simulink model "humanFollower1"  (R2018b)
settings: Solver=VariableStepAuto  StartTime=0.0  StopTime=inf  MaxStep=0.2  MinStep=0.2  RelTol=1e-3
undefined symbols (not defined in the file or in its folder): Angular, Linear
libraries: robotlib x8
settings Model: Creator=ckreienk  LastModifiedBy=ckreienk
settings SolverCC: InitialStep=0.2

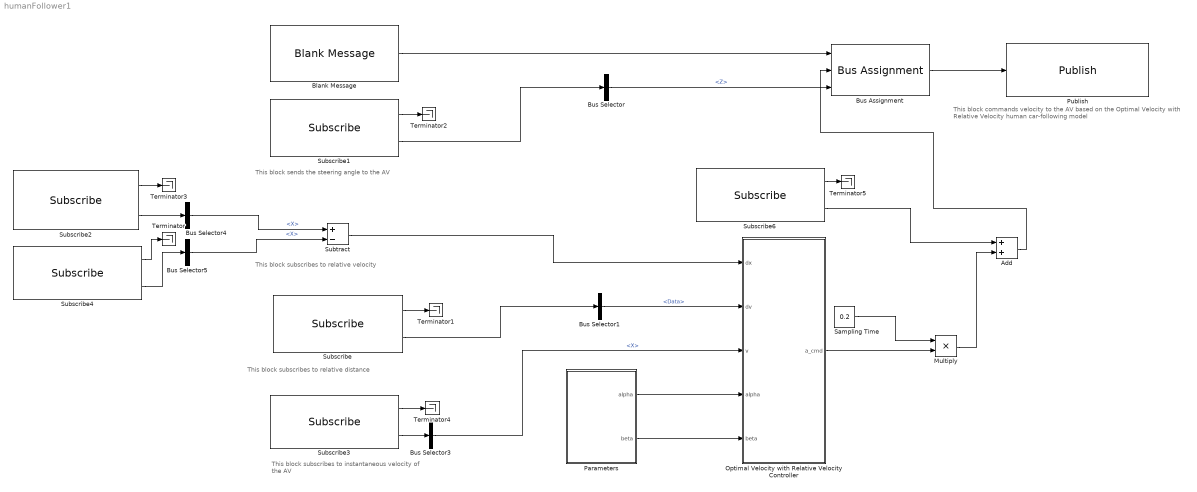
== system humanFollower1 ==
  note: This block sends the steering angle
      | to the AV
  note: This block subscribes to relative velocity
  note: This block subscribes to relative distance
  note: This block subscribes to
      | instantaneous velocity of the AV
  note: This block commands velocity to the AV based
      | on the Optimal Velocity with Relative Velocity
      | human car-following model
  Add : Sum
  Blank Message : robotlib/Blank Message  messageClass=Message  entityType=geometry_msgs/Twist  messageType=geometry_msgs/Twist  SampleTime=inf
      settings: SourceProductBaseCode=RO
  Bus Assignment : BusAssignment  AssignedSignals=Linear.X,Angular.Z
  Bus Selector : BusSelector  OutputSignals=Angular.Z
  Bus Selector1 : BusSelector  OutputSignals=Data
  Bus Selector3 : BusSelector  OutputSignals=Linear.X
  Bus Selector4 : BusSelector  OutputSignals=Linear.X
  Bus Selector5 : BusSelector  OutputSignals=Linear.X
  Multiply : Product
  Optimal Velocity with Relative Velocity Controller : Subsystem
  Parameters : Subsystem
  Publish : robotlib/Publish  topicSource=Select from ROS network  topic=/followerVehicle/cmd_vel  messageType=geometry_msgs/Twist  messageQueueLength=1
      settings: SourceProductBaseCode=RO
  Sampling Time : Constant  Value=0.2
  Subscribe : robotlib/Subscribe  topicSource=Select from ROS network  topic=/followerVehicle/distanceEstimatorSteeringBased/dist  messageType=std_msgs/Float64  sampleTime=-1  messageQueueLength=1
      settings: SourceProductBaseCode=RO
  Subscribe1 : robotlib/Subscribe  topicSource=Select from ROS network  topic=/leadVehicle/cmd_vel  messageType=geometry_msgs/Twist  sampleTime=-1  messageQueueLength=1
      settings: SourceProductBaseCode=RO
  Subscribe2 : robotlib/Subscribe  topicSource=Select from ROS network  topic=/leadVehicle/cmd_vel  messageType=geometry_msgs/Twist  sampleTime=-1  messageQueueLength=1
      settings: SourceProductBaseCode=RO
  Subscribe3 : robotlib/Subscribe  topicSource=Select from ROS network  topic=/followerVehicle/cmd_vel  messageType=geometry_msgs/Twist  sampleTime=-1  messageQueueLength=1
      settings: SourceProductBaseCode=RO
  Subscribe4 : robotlib/Subscribe  topicSource=Select from ROS network  topic=/followerVehicle/cmd_vel  messageType=geometry_msgs/Twist  sampleTime=-1  messageQueueLength=1
      settings: SourceProductBaseCode=RO
  Subscribe6 : robotlib/Subscribe  topicSource=Select from ROS network  topic=/followerVehicle/cmd_vel  messageType=geometry_msgs/Twist  sampleTime=-1  messageQueueLength=1
      settings: SourceProductBaseCode=RO
  Subtract : Sum  Inputs=+-
  Terminator{,1..5} (6 alike) : Terminator
  wires:
  Bus Selector5/1 -> Subtract/2  "<X>"
  Subscribe4/2 -> Bus Selector5/1
  Bus Selector4/1 -> Subtract/1  "<X>"
  Subscribe2/2 -> Bus Selector4/1
  Subtract/1 -> Optimal Velocity with Relative Velocity Controller/1(dx)
  Subscribe4/1 -> Terminator/1
  Parameters/2(beta) -> Optimal Velocity with Relative Velocity Controller/5(beta)
  Parameters/1(alpha) -> Optimal Velocity with Relative Velocity Controller/4(alpha)
  Bus Selector/1 -> Bus Assignment/3  "<Z>"
  Bus Selector3/1 -> Optimal Velocity with Relative Velocity Controller/3(v)  "<X>"
  Bus Selector1/1 -> Optimal Velocity with Relative Velocity Controller/2(dv)  "<Data>"
  Subscribe3/2 -> Bus Selector3/1
  Subscribe3/1 -> Terminator4/1
  Subscribe2/1 -> Terminator3/1
  Subscribe1/1 -> Terminator2/1
  Subscribe/2 -> Bus Selector1/1
  Subscribe/1 -> Terminator1/1
  Bus Assignment/1 -> Publish/1
  Blank Message/1 -> Bus Assignment/1
  Subscribe1/2 -> Bus Selector/1
  Subscribe6/1 -> Terminator5/1
  Add/1 -> Bus Assignment/2
  Optimal Velocity with Relative Velocity Controller/1(a_cmd) -> Multiply/2
  Sampling Time/1 -> Multiply/1
  Multiply/1 -> Add/2
  Subscribe6/2 -> Add/1

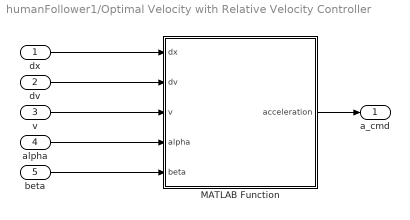
== system humanFollower1/Optimal Velocity with Relative Velocity Controller ==
  dx : Inport
  dv : Inport  Port=2
  v : Inport  Port=3
  alpha : Inport  Port=4
  beta : Inport  Port=5
  MATLAB Function : MATLAB Function  TreatAsAtomicUnit=on
  a_cmd : Outport
  wires:
  MATLAB Function/1(acceleration) -> a_cmd/1
  dx/1 -> MATLAB Function/1(dx)
  dv/1 -> MATLAB Function/2(dv)
  v/1 -> MATLAB Function/3(v)
  alpha/1 -> MATLAB Function/4(alpha)
  beta/1 -> MATLAB Function/5(beta)

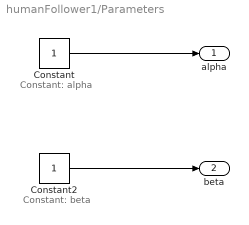
== system humanFollower1/Parameters ==
  note: Constant: beta
  note: Constant: alpha
  Constant : Constant
  Constant2 : Constant
  alpha : Outport
  beta : Outport  Port=2
  wires:
  Constant/1 -> alpha/1
  Constant2/1 -> beta/1

== matlab function humanFollower1/Optimal Velocity with Relative Velocity Controller/MATLAB Function ==
  data: dx input; dv input; v input; alpha input; acceleration output; beta input
function acceleration = fcn(dx, dv, v, alpha, beta)
eqSpeedSpacing = dx*3;
acceleration = alpha*(eqSpeedSpacing - v) + beta*dv
